simulink library "dq_to_alpha_beta"  (R2026a)
settings: Solver=VariableStepAuto
settings Model: Creator=dbagn  LastModifiedBy=dbagn

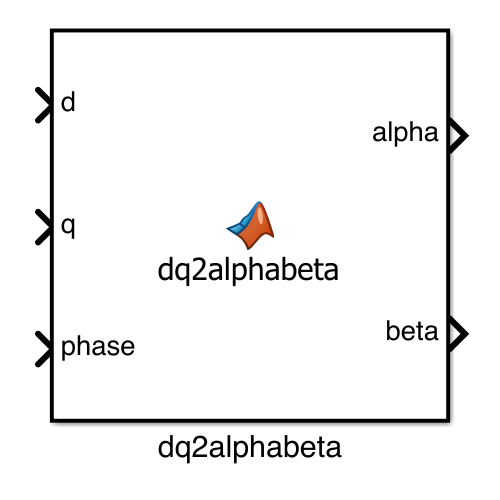
[thumbnail: Simulink's stored preview of the top-level diagram]
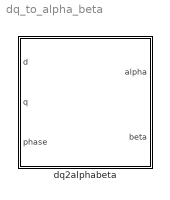
== system dq_to_alpha_beta ==
  dq2alphabeta : MATLAB Function  TreatAsAtomicUnit=on

== matlab function dq_to_alpha_beta/dq2alphabeta ==
  data: d input; alpha output; q input; phase input; beta output
function [alpha,beta] = dq2alphabeta(d,q,phase)

    alpha  =  d*cos(phase) - q*sin(phase);
    beta = d*sin(phase) + q*cos(phase);

end
